simulink model "VELOmodel_i2pacl_steps"  (R2021b)
settings: Solver=ode23t  StartTime=0  StopTime=15000  FixedStep=0.001  MaxStep=0.1  RelTol=1e-6  AbsTol=1e-3  EnableMultiTasking=on
values from neighbouring files (symbols this model uses):
  CO2PropertyTables =     [CO2properties.mat]
  I_conductivity = 0.033    [simscape_paramaters_testing.m]
  initTemp = 20+273.15    (= 293.15)    [simscape_paramaters_testing.m]
  pump_volume = 9.5e-6    (= 9.5e-06)    [simscape_paramaters_testing.m]
  quater_diameter = 6.35/1000    (= 0.00635)    [simscape_paramaters_testing.m]
  quater_wall_thickness = 0.89/1000    (= 0.00089)    [simscape_paramaters_testing.m]
  SS_density = 8000    [simscape_paramaters_testing.m]
  swep_length = swep_area/(2*pi*swep_radius)    (= 6868.79228081)    [simscape_paramaters_testing.m]
  swep_radius = 3.8    [simscape_paramaters_testing.m]
  T_ambient = 273.15+20    (= 293.15)    [simscape_paramaters_testing.m]
  t_start = 3000+t_cool    (= 5000)    [simscape_paramaters_testing.m]
  TL_length = 10    [simscape_paramaters_testing.m]
  TL_supply_diameter = 0.005    [simscape_paramaters_testing.m]
libraries: fl_lib x99, nesl_utility x20, SimscapeFluids_lib x1, slpidlib x1
(part 2 of 2)

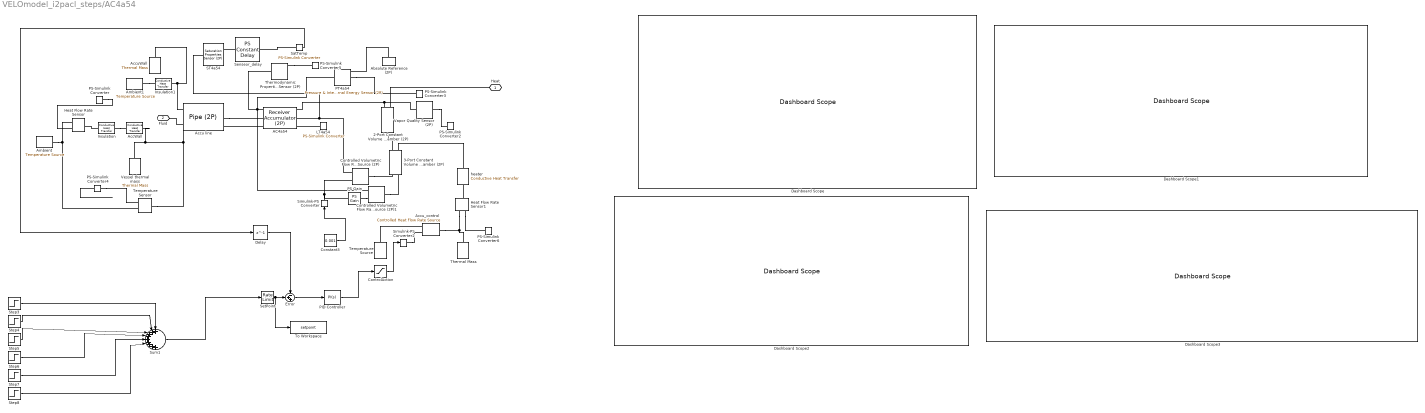
== system VELOmodel_i2pacl_steps/AC4a54 ==
  2-Port Constant Volume Chamber (2P) : fl_lib/Two-Phase Fluid/Elements/2-Port Constant Volume Chamber (2P)  volume=1 l  area_A=1 m^2  area_B=1 m^2  energy_spec=foundation.enum.energy_spec.void_fraction  p_init=initPressure MPa  T_init=initTemp K  x_init=0.5  alpha_init=0.7  h_init=1500 kJ/kg  u_init=1500 kJ/kg  time_constant=0.1 s
      settings: SourceProductBaseCode=SS  InternalSimscapePortConfiguration="{\"Bottom\":[],\"Left\":[{\"id\":\"A\",\"label\":\"A\",\"type\":\"foundation.two_phase_fluid.two_phase_fluid\"},{\"id\":\"H\",\"label\":\"H\",\"type\":\"foundation.thermal.thermal\"}],\"Right\":[{\"id\":\"B\",\"label\":\"B\",\"type\":\"foundation.two_phase_fluid.two_phase_fluid\"}],\"Top\":[]}"
  3-Port Constant Volume Chamber (2P) : fl_lib/Two-Phase Fluid/Elements/3-Port Constant Volume Chamber (2P)  volume=2 l  area_A=1 m^2  area_B=1 m^2  area_C=1 m^2  energy_spec=foundation.enum.energy_spec.void_fraction  p_init=initPressure MPa  T_init=initTemp K  x_init=0.5  alpha_init=0.7  h_init=1500 kJ/kg  u_init=1500 kJ/kg  time_constant=0.1 s
      settings: SourceProductBaseCode=SS  InternalSimscapePortConfiguration="{\"Bottom\":[],\"Left\":[{\"id\":\"A\",\"label\":\"A\",\"type\":\"foundation.two_phase_fluid.two_phase_fluid\"},{\"id\":\"H\",\"label\":\"H\",\"type\":\"foundation.thermal.thermal\"}],\"Right\":[{\"id\":\"B\",\"label\":\"B\",\"type\":\"foundation.two_phase_fluid.two_phase_fluid\"},{\"id\":\"C\",\"label\":\"C\",\"type\":\"foundation.two_phase_fluid.two_phase_fluid\"}],\"Top\":[]}"
  AC4a54 : SimscapeFluids_lib/Two-Phase Fluid/Tanks & Accumulators/Receiver Accumulator (2P)  volume=Acc_volume l  area_AV=1 m^2  area_BV=1 m^2  area_AL=quater_area m^2  area_BL=1 m^2  V_frac_error=simscape.enum.assert.action.none  V_frac_min=0.05  V_frac_max=0.95  V_frac_smooth=0.05  p_crit_error=simscape.enum.assert.action.warn  hc_vap=20 W/(m^2*K)  hc_liq=100 W/(m^2*K)  surface_area=0.5 m^2  receiver_accumulator_energy_spec=fluids.two_phase_fluid.enum.receiver_accumulator_energy_spec.volume_fraction  p_init=initPressure MPa  T_init=initTemp K  M_frac_init=0.5  V_frac_init=0.3  h_init=1500 kJ/kg  u_init=1500 kJ/kg  tau_vap_cond=1 s
      settings: SourceProductBaseCode=SH  InternalSimscapePortConfiguration="{\"Bottom\":[],\"Left\":[{\"id\":\"AV\",\"label\":\"AV\",\"type\":\"foundation.two_phase_fluid.two_phase_fluid\"},{\"id\":\"AL\",\"label\":\"AL\",\"type\":\"foundation.two_phase_fluid.two_phase_fluid\"},{\"id\":\"H\",\"label\":\"H\",\"type\":\"foundation.thermal.thermal\"}],\"Right\":[{\"id\":\"BV\",\"label\":\"BV\",\"type\":\"foundation.two_phase_fluid.two_phase_fluid\"},{\"id\":\"BL\",\"label\":\"BL\",\"type\":\"foundation.two_phase_fluid.two_phase_fluid\"},{\"id\":\"L\",\"label\":\"L\",\"type\":\"output\"}],\"Top\":[]}"
  Absolute Reference (2P) : fl_lib/Two-Phase Fluid/Elements/Absolute Reference (2P)
      settings: SourceProductBaseCode=SS
  AccWall : fl_lib/Thermal/Thermal Elements/Conductive Heat Transfer  area=I_area m^2  thickness=Acc_thickness m  th_cond=SS_conductivity W/(m*K)  T_specify=off  T_priority=None  T=0 K  T_nominal_specify=off  T_nominal_unit=K  T_nominal_value=1  Q_specify=off  Q_priority=None  Q=0 W  Q_nominal_specify=off  Q_nominal_unit=W  Q_nominal_value=1
  Accu line : fl_lib/Two-Phase Fluid/Elements/Pipe (2P)  length=0.5 m  area=quater_area m^2  Dh=quater_diameter m  length_add=0.1 m  roughness=15e-6 m  Re_lam=2000  Re_tur=4000  shape_factor=64  Nu_lam=3.66  inertia=simscape.enum.onoff.off  energy_spec=foundation.enum.energy_spec.void_fraction  p_init=initPressure MPa  T_init=initTemp K  x_init=0  alpha_init=voidFrac  h_init=1500 kJ/kg  u_init=1500 kJ/kg  mdot_init=0 kg/s  time_constant=0.1 s
      settings: SourceProductBaseCode=SS  InternalSimscapePortConfiguration="{\"Bottom\":[],\"Left\":[{\"id\":\"A\",\"label\":\"A\",\"type\":\"foundation.two_phase_fluid.two_phase_fluid\"},{\"id\":\"H\",\"label\":\"H\",\"type\":\"foundation.thermal.thermal\"}],\"Right\":[{\"id\":\"B\",\"label\":\"B\",\"type\":\"foundation.two_phase_fluid.two_phase_fluid\"}],\"Top\":[]}"
  AccuWall : fl_lib/Thermal/Thermal Elements/Thermal Mass  mass=0.5 kg  sp_heat=SS_specific_heat J/(K*kg)  T_specify=on  T_priority=High  T=initTemp K  T_nominal_specify=off  T_nominal_unit=K  T_nominal_value=1  Q_specify=off  Q_priority=None  Q=0 W  Q_nominal_specify=off  Q_nominal_unit=W  Q_nominal_value=1
  Accu_control : fl_lib/Thermal/Thermal Sources/Controlled Heat Flow Rate Source
  Ambient : fl_lib/Thermal/Thermal Sources/Temperature Source  temperature=T_ambient K
  Ambient1 : fl_lib/Thermal/Thermal Sources/Temperature Source  temperature=T_ambient K
  Constant3 : Constant  Value=0.001
  ControlAction : Saturate  UpperLimit=1000  LowerLimit=-1000
  Controlled Volumetric Flow Rate Source (2P) : fl_lib/Two-Phase Fluid/Sources/Controlled Volumetric Flow Rate Source (2P)  power_spec=foundation.enum.power_spec.none  area_A=1 m^2  area_B=1 m^2
      settings: SourceProductBaseCode=SS  InternalSimscapePortConfiguration="{\"Bottom\":[],\"Left\":[{\"id\":\"A\",\"label\":\"A\",\"type\":\"foundation.two_phase_fluid.two_phase_fluid\"},{\"id\":\"V\",\"label\":\"V\",\"type\":\"input\"}],\"Right\":[{\"id\":\"B\",\"label\":\"B\",\"type\":\"foundation.two_phase_fluid.two_phase_fluid\"}],\"Top\":[]}"
  Controlled Volumetric Flow Rate Source (2P)1 : fl_lib/Two-Phase Fluid/Sources/Controlled Volumetric Flow Rate Source (2P)  power_spec=foundation.enum.power_spec.none  area_A=1 m^2  area_B=1 m^2
      settings: SourceProductBaseCode=SS  InternalSimscapePortConfiguration="{\"Bottom\":[],\"Left\":[{\"id\":\"A\",\"label\":\"A\",\"type\":\"foundation.two_phase_fluid.two_phase_fluid\"},{\"id\":\"V\",\"label\":\"V\",\"type\":\"input\"}],\"Right\":[{\"id\":\"B\",\"label\":\"B\",\"type\":\"foundation.two_phase_fluid.two_phase_fluid\"}],\"Top\":[]}"
  Dashboard Scope{,1..3} (4 alike) : DashboardScope
  Delay : Delay  DelayLength=1  InitialCondition=initTemp+5.35
  Error : Sum  Inputs=-++
  Heat Flow Rate Sensor : fl_lib/Thermal/Thermal Sensors/Heat Flow Rate Sensor
      settings: SourceProductBaseCode=SS
  Heat Flow Rate Sensor1 : fl_lib/Thermal/Thermal Sensors/Heat Flow Rate Sensor
      settings: SourceProductBaseCode=SS
  Insulation : fl_lib/Thermal/Thermal Elements/Conductive Heat Transfer  area=I_area m^2  thickness=I_thickness m  th_cond=I_conductivity*4 W/(m*K)  T_specify=off  T_priority=None  T=0 K  T_nominal_specify=off  T_nominal_unit=K  T_nominal_value=1  Q_specify=off  Q_priority=None  Q=0 W  Q_nominal_specify=off  Q_nominal_unit=W  Q_nominal_value=1
  Insulation1 : fl_lib/Thermal/Thermal Elements/Conductive Heat Transfer  area=pi*quater_diameter*1 m^2  thickness=I_thickness m  th_cond=I_conductivity W/(m*K)  T_specify=off  T_priority=None  T=0 K  T_nominal_specify=off  T_nominal_unit=K  T_nominal_value=1  Q_specify=off  Q_priority=None  Q=0 W  Q_nominal_specify=off  Q_nominal_unit=W  Q_nominal_value=1
  LT4a54 : nesl_utility/PS-Simulink Converter  PhysicalDomain=network_engine_domain  SubClassName=ps_output  LeftPortType=input  RightPortType=output  PseudoPeriodic=off  Frequencies=[]  Unit=inherit  AffineConversion=off
      settings: SourceProductBaseCode=PW,SS
  PID Controller : slpidlib/PID Controller  Controller=PI  Form=Ideal  TimeDomain=Continuous-time  UseExternalTs=off  SampleTime=-1  IntegratorMethod=Forward Euler  FilterMethod=Forward Euler  ControllerParametersSource=internal  P=711  I=1/186  D=0  UseFilter=on  N=100  TunerSelectOption=Transfer Function Based (PID Tuner App)  InitialConditionSource=internal  InitialConditionForIntegrator=0  InitialConditionForFilter=0  DifferentiatorICPrevScaledInput=0  ExternalReset=none  TrackingMode=off  Kt=1  LimitOutput=on  SatLimitsSource=internal  UpperSaturationLimit=1000  LowerSaturationLimit=-1000  LinearizeAsGain=on  AntiWindupMode=clamping  Kb=1  POutMin=[]  POutMax=[]  IOutMin=[]  IOutMax=[]  DOutMin=[]  DOutMax=[]  NOutMin=[]  NOutMax=[]  SumOutMin=[]  SumOutMax=[]  SaturationOutMin=[]  SaturationOutMax=[]  PParamMin=[]  PParamMax=[]  IParamMin=[]  IParamMax=[]  DParamMin=[]  DParamMax=[]  NParamMin=[]  NParamMax=[]  KbParamMin=[]  KbParamMax=[]  KtParamMin=[]  KtParamMax=[]  KbOutMin=[]  KbOutMax=[]  KtOutMin=[]  KtOutMax=[]  IntegratorOutMin=[]  IntegratorOutMax=[]  FilterOutMin=[]  FilterOutMax=[]  SumI1OutMin=[]  SumI1OutMax=[]  SumI2OutMin=[]  SumI2OutMax=[]  SumI3OutMin=[]  SumI3OutMax=[]  SumI4OutMin=[]  SumI4OutMax=[]  SumDOutMin=[]  SumDOutMax=[]  DifferentiatorOutMin=[]  DifferentiatorOutMax=[]  FilterDiffOutCoefMin=[]  FilterDiffOutCoefMax=[]  ReciprocalOutMin=[]  ReciprocalOutMax=[]  SumDenOutMin=[]  SumDenOutMax=[]  SumNumOutMin=[]  SumNumOutMax=[]  DivideOutMin=[]  DivideOutMax=[]  UdiffTsProdOutMin=[]  UdiffTsProdOutMax=[]  NTsProdOutMin=[]  NTsProdOutMax=[]  UintegralTsProdOutMin=[]  UintegralTsProdOutMax=[]  UngainTsProdOutMin=[]  UngainTsProdOutMax=[]  IntegratorContinuousStateAttributes=''  IntegratorStateMustResolveToSignalObject=off  IntegratorRTWStateStorageClass=Auto  FilterContinuousStateAttributes=''  FilterStateMustResolveToSignalObject=off  FilterRTWStateStorageClass=Auto  ParallelPVariant=Passthrough  IdealPVariant=InternalParameters  IVariant=InternalParameters  DVariant=Disabled  IntegratorVariant=Continuous  SatVariant=Enabled  AWVariant=ContClampingIdeal  PCopyVariant=InternalParamsIdeal  TRVariant=Disabled  FdbkBlocksVariant=Forward  IdealPFdbkVariant=Disabled  SatFdbkVariant=Disabled  DerivativeFilterVariant=Disabled  NVariant=Disabled  NCopyVariant=Disabled_SignalSpec  FilterICVariant=Disabled  IntegratorICVariant=InternalICs  ExternalResetVariant=Disabled  TRSumVariant=Passthrough  SumFdbkVariant=Disabled  SumVariant=Sum_PI  TsampFilterVariant=InternalTs  TsampNgainVariant=Passthrough  TsampIntegralVariant=Passthrough  ExternalSaturationOutDataTypeStr=Inherit: Same as second input
  PS Gain : fl_lib/Physical Signals/Functions/PS Gain  gain=10
  PS-Simulink Converter{,2..6} (6 alike) : nesl_utility/PS-Simulink Converter  PhysicalDomain=network_engine_domain  SubClassName=ps_output  LeftPortType=input  RightPortType=output  PseudoPeriodic=off  Frequencies=[]  Unit=inherit  AffineConversion=off
      settings: SourceProductBaseCode=PW,SS
  PT4a54 : fl_lib/Two-Phase Fluid/Sensors/Pressure & Internal Energy Sensor (2P)
      settings: SourceProductBaseCode=SS  InternalSimscapePortConfiguration="{\"Bottom\":[],\"Left\":[{\"id\":\"A\",\"label\":\"A\",\"type\":\"foundation.two_phase_fluid.two_phase_fluid\"}],\"Right\":[{\"id\":\"B\",\"label\":\"B\",\"type\":\"foundation.two_phase_fluid.two_phase_fluid\"},{\"id\":\"P\",\"label\":\"P\",\"type\":\"output\"},{\"id\":\"U\",\"label\":\"U\",\"type\":\"output\"}],\"Top\":[]}"
  ST4a54 : fl_lib/Two-Phase Fluid/Sensors/Saturation Properties Sensor (2P)  pressure_measure=simscape.enum.onoff.off  pressure_check=simscape.enum.assert.action.error  energy_measure=foundation.enum.EnergyMeasurement.Off  density_measure=foundation.enum.DensityMeasurement.Off
      settings: SourceProductBaseCode=SS  InternalSimscapePortConfiguration="{\"Bottom\":[],\"Left\":[{\"id\":\"A\",\"label\":\"A\",\"type\":\"foundation.two_phase_fluid.two_phase_fluid\"}],\"Right\":[{\"id\":\"T_sat_liq\",\"label\":\"TL\",\"type\":\"output\"},{\"id\":\"T_sat_vap\",\"label\":\"TV\",\"type\":\"output\"}],\"Top\":[]}"
  SatTemp : nesl_utility/PS-Simulink Converter  PhysicalDomain=network_engine_domain  SubClassName=ps_output  LeftPortType=input  RightPortType=output  PseudoPeriodic=off  Frequencies=[]  Unit=inherit  AffineConversion=off
      settings: SourceProductBaseCode=PW,SS
  Senseor_delay : fl_lib/Physical Signals/Delays/PS Constant Delay  InputHistory=initTemp K  DelayTime=55 ms
      settings: SourceProductBaseCode=SS  InternalSimscapePortConfiguration="{\"Bottom\":[],\"Left\":[{\"id\":\"U\",\"label\":\"U\",\"type\":\"input\"}],\"Right\":[{\"id\":\"Y\",\"label\":\"Y\",\"type\":\"output\"}],\"Top\":[]}"
  SetPoint : RateLimiter  RisingSlewLimit=1.333/60  FallingSlewLimit=-1.333/60  SampleTimeMode=inherited
  Simulink-PS Converter : nesl_utility/Simulink-PS Converter  PhysicalDomain=network_engine_domain  SubClassName=ps_input  LeftPortType=input  RightPortType=output  PseudoPeriodic=off  Frequencies=[]  NoiseDistribution=none  NoiseParameters=[]  Unit=1  AffineConversion=off  FilteringAndDerivatives=provide  SimscapeFilterOrder=1  InputFilterTimeConstant=0.001  UdotUserProvided=0
      settings: SourceProductBaseCode=PW,SS
  Simulink-PS Converter2 : nesl_utility/Simulink-PS Converter  PhysicalDomain=network_engine_domain  SubClassName=ps_input  LeftPortType=input  RightPortType=output  PseudoPeriodic=off  Frequencies=[]  NoiseDistribution=none  NoiseParameters=[]  Unit=1  AffineConversion=off  FilteringAndDerivatives=provide  SimscapeFilterOrder=1  InputFilterTimeConstant=0.001  UdotUserProvided=0
      settings: SourceProductBaseCode=PW,SS
  Step3 : Step  Time=500  Before=initTemp  After=273.15-25  SampleTime=0
  Step4 : Step  Time=5000  After=10  SampleTime=0
  Step5 : Step  Time=7000  After=10  SampleTime=0
  Step6 : Step  Time=9000  After=10  SampleTime=0
  Step7 : Step  Time=11000  After=10  SampleTime=0
  Step8 : Step  Time=13000  After=10  SampleTime=0
  Sum1 : Sum  Inputs=+++++++++
  Temperature Sensor : fl_lib/Thermal/Thermal Sensors/Temperature Sensor
  Temperature Source : fl_lib/Thermal/Thermal Sources/Temperature Source  temperature=273 K
  Thermal Mass : fl_lib/Thermal/Thermal Elements/Thermal Mass  mass=2 kg  sp_heat=SS_specific_heat J/(K*kg)  T_specify=on  T_priority=High  T=initTemp K  T_nominal_specify=off  T_nominal_unit=K  T_nominal_value=1  Q_specify=off  Q_priority=None  Q=0 W  Q_nominal_specify=off  Q_nominal_unit=W  Q_nominal_value=1
  Thermodynamic Properties Sensor (2P) : fl_lib/Two-Phase Fluid/Sensors/Thermodynamic Properties Sensor (2P)
      settings: SourceProductBaseCode=SS  InternalSimscapePortConfiguration="{\"Bottom\":[],\"Left\":[{\"id\":\"A\",\"label\":\"A\",\"type\":\"foundation.two_phase_fluid.two_phase_fluid\"}],\"Right\":[{\"id\":\"T\",\"label\":\"T\",\"type\":\"output\"},{\"id\":\"H\",\"label\":\"h\",\"type\":\"output\"},{\"id\":\"V\",\"label\":\"v\",\"type\":\"output\"},{\"id\":\"S\",\"label\":\"s\",\"type\":\"output\"}],\"Top\":[]}"
  To Workspace : ToWorkspace  VariableName=setpoint  SaveFormat=Timeseries  SampleTime=-1
  Vapor Quality Sensor (2P) : fl_lib/Two-Phase Fluid/Sensors/Vapor Quality Sensor (2P)  vapor_fraction_spec=foundation.enum.vapor_fraction_spec.quality
      settings: SourceProductBaseCode=SS  InternalSimscapePortConfiguration="{\"Bottom\":[],\"Left\":[{\"id\":\"A\",\"label\":\"A\",\"type\":\"foundation.two_phase_fluid.two_phase_fluid\"}],\"Right\":[{\"id\":\"X\",\"label\":\"X\",\"type\":\"output\"}],\"Top\":[]}"
  Vessel thermal mass : fl_lib/Thermal/Thermal Elements/Thermal Mass  mass=A_mass kg  sp_heat=SS_specific_heat J/(K*kg)  T_specify=on  T_priority=High  T=initTemp K  T_nominal_specify=off  T_nominal_unit=K  T_nominal_value=1  Q_specify=off  Q_priority=None  Q=0 W  Q_nominal_specify=off  Q_nominal_unit=W  Q_nominal_value=1
  heater : fl_lib/Thermal/Thermal Elements/Conductive Heat Transfer  area=0.25 m^2  thickness=0.001 m  th_cond=SS_conductivity W/(m*K)  T_specify=off  T_priority=None  T=0 K  T_nominal_specify=off  T_nominal_unit=K  T_nominal_value=1  Q_specify=off  Q_priority=None  Q=0 W  Q_nominal_specify=off  Q_nominal_unit=W  Q_nominal_value=1
  Heat : PMIOPort  Side=Left
  Fluid : PMIOPort  Port=2  Side=Left
  wires:
  PS-Simulink Converter4/1 -> ?
  SatTemp/1 -> Delay/1
  Constant3/1 -> Simulink-PS Converter/1
  PID Controller/1 -> ControlAction/1
  SetPoint/1 -> To Workspace/1, Error/2
  Error/1 -> PID Controller/1
  Delay/1 -> Error/1
  ControlAction/1 -> Simulink-PS Converter2/1
  Step8/1 -> Sum1/6
  Step7/1 -> Sum1/5
  Step5/1 -> Sum1/3
  Step4/1 -> Sum1/2
  Step6/1 -> Sum1/4
  Sum1/1 -> SetPoint/1
  Step3/1 -> Sum1/1
  connections:
  Vessel thermal mass/LConn1 -- AccWall/RConn1 -- Temperature Sensor/LConn1 -- AC4a54/LConn3
  LT4a54/LConn1 -- AC4a54/RConn3
  AC4a54/LConn1 -- Thermodynamic Properties Sensor (2P)/LConn1 -- PT4a54/LConn1 -- Controlled Volumetric Flow Rate Source (2P)1/LConn1
  Temperature Source/LConn1 -- Accu_control/RConn2
  Vapor Quality Sensor (2P)/RConn1 -- PS-Simulink Converter2/LConn1
  Vapor Quality Sensor (2P)/LConn1 -- 2-Port Constant Volume Chamber (2P)/LConn1 -- AC4a54/RConn1
  Absolute Reference (2P)/LConn1 -- PT4a54/RConn1
  PT4a54/RConn2 -- PS-Simulink Converter3/LConn1
  Controlled Volumetric Flow Rate Source (2P)/LConn1 -- ST4a54/LConn1 -- AC4a54/RConn2
  Controlled Volumetric Flow Rate Source (2P)/LConn2 -- PS Gain/LConn1 -- Simulink-PS Converter/RConn1
  Senseor_delay/LConn1 -- ST4a54/RConn1
  Temperature Sensor/RConn1 -- Ambient/LConn1 -- Heat Flow Rate Sensor/RConn2
  PS-Simulink Converter/LConn1 -- Heat Flow Rate Sensor/RConn1
  PS-Simulink Converter4/LConn1 -- Temperature Sensor/RConn2
  Thermodynamic Properties Sensor (2P)/RConn1 -- PS-Simulink Converter5/LConn1
  Heat Flow Rate Sensor1/RConn2 -- Accu_control/LConn1 -- Thermal Mass/LConn1
  3-Port Constant Volume Chamber (2P)/LConn2 -- heater/RConn1
  Heat Flow Rate Sensor1/LConn1 -- heater/LConn1
  Heat Flow Rate Sensor1/RConn1 -- PS-Simulink Converter6/LConn1
  Simulink-PS Converter2/RConn1 -- Accu_control/RConn1
  Controlled Volumetric Flow Rate Source (2P)/RConn1 -- 3-Port Constant Volume Chamber (2P)/RConn1
  Controlled Volumetric Flow Rate Source (2P)1/RConn1 -- 3-Port Constant Volume Chamber (2P)/RConn2
  PS Gain/RConn1 -- Controlled Volumetric Flow Rate Source (2P)1/LConn2
  3-Port Constant Volume Chamber (2P)/LConn1 -- 2-Port Constant Volume Chamber (2P)/RConn1
  Heat/RConn1 -- 2-Port Constant Volume Chamber (2P)/LConn2
  SatTemp/LConn1 -- Senseor_delay/RConn1
  Accu line/RConn1 -- AC4a54/LConn2
  Accu line/LConn1 -- Fluid/RConn1
  Ambient1/LConn1 -- Insulation1/LConn1
  Insulation1/RConn1 -- AccuWall/LConn1 -- Accu line/LConn2
  Insulation/RConn1 -- AccWall/LConn1
  Insulation/LConn1 -- Heat Flow Rate Sensor/LConn1

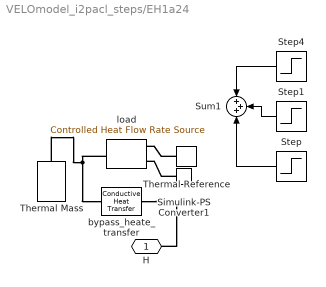
== system VELOmodel_i2pacl_steps/EH1a24 ==
  Simulink-PS Converter1 : nesl_utility/Simulink-PS Converter  PhysicalDomain=network_engine_domain  SubClassName=ps_input  LeftPortType=input  RightPortType=output  PseudoPeriodic=off  Frequencies=[]  NoiseDistribution=none  NoiseParameters=[]  Unit=1  AffineConversion=off  FilteringAndDerivatives=provide  SimscapeFilterOrder=1  InputFilterTimeConstant=0.001  UdotUserProvided=0
      settings: SourceProductBaseCode=PW,SS
  Step : Step  Time=t_start+140  After=400  SampleTime=0
  Step1 : Step  Time=t_start  After=110  SampleTime=0
  Step4 : Step  Time=t_start+5130  After=-510  SampleTime=0
  Sum1 : Sum  Inputs=+++
  Thermal Mass : fl_lib/Thermal/Thermal Elements/Thermal Mass  mass=10 kg  sp_heat=SS_specific_heat J/(K*kg)  T_specify=on  T_priority=High  T=initTemp K  T_nominal_specify=off  T_nominal_unit=K  T_nominal_value=1  Q_specify=off  Q_priority=None  Q=0 W  Q_nominal_specify=off  Q_nominal_unit=W  Q_nominal_value=1
  Thermal Reference : fl_lib/Thermal/Thermal Elements/Thermal Reference
  bypass_heate_transfer : fl_lib/Thermal/Thermal Elements/Conductive Heat Transfer  area=0.25 m^2  thickness=0.001 m  th_cond=SS_conductivity W/(m*K)  T_specify=off  T_priority=None  T=0 K  T_nominal_specify=off  T_nominal_unit=K  T_nominal_value=1  Q_specify=off  Q_priority=None  Q=0 W  Q_nominal_specify=off  Q_nominal_unit=W  Q_nominal_value=1
  load : fl_lib/Thermal/Thermal Sources/Controlled Heat Flow Rate Source
  H : PMIOPort  Side=Right
  wires:
  Step1/1 -> Sum1/2
  Step4/1 -> Sum1/1
  Step/1 -> Sum1/3
  connections:
  Simulink-PS Converter1/RConn1 -- load/RConn1
  load/LConn1 -- Thermal Mass/LConn1 -- bypass_heate_transfer/LConn1
  Thermal Reference/LConn1 -- load/RConn2
  bypass_heate_transfer/RConn1 -- H/RConn1

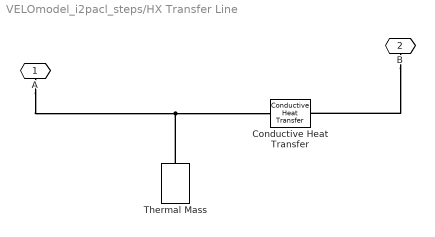
== system VELOmodel_i2pacl_steps/HX Transfer Line ==
  Conductive Heat Transfer : fl_lib/Thermal/Thermal Elements/Conductive Heat Transfer  area=TL_length*pi*TL_supply_diameter m^2  thickness=TL_wall_thickness m  th_cond=SS_conductivity W/(m*K)  T_specify=off  T_priority=None  T=0 K  T_nominal_specify=off  T_nominal_unit=K  T_nominal_value=1  Q_specify=off  Q_priority=None  Q=0 W  Q_nominal_specify=off  Q_nominal_unit=W  Q_nominal_value=1
  Thermal Mass : fl_lib/Thermal/Thermal Elements/Thermal Mass  mass=TL_length*pi*quater_diameter*quater_wall_thickness*SS_density kg  sp_heat=SS_specific_heat J/(K*kg)  T_specify=off  T_priority=High  T=300 K  T_nominal_specify=off  T_nominal_unit=K  T_nominal_value=1  Q_specify=off  Q_priority=None  Q=0 W  Q_nominal_specify=off  Q_nominal_unit=W  Q_nominal_value=1
  A : PMIOPort  Side=Left
  B : PMIOPort  Port=2  Side=Right
  connections:
  B/RConn1 -- Conductive Heat Transfer/RConn1
  A/RConn1 -- Conductive Heat Transfer/LConn1 -- Thermal Mass/LConn1

== system VELOmodel_i2pacl_steps/HX4a54b ==
  Conductive Heat Transfer : fl_lib/Thermal/Thermal Elements/Conductive Heat Transfer  area=hx_sa m^2  thickness=quater_wall_thickness m  th_cond=SS_conductivity W/(m*K)  T_specify=off  T_priority=None  T=0 K  T_nominal_specify=off  T_nominal_unit=K  T_nominal_value=1  Q_specify=off  Q_priority=None  Q=0 W  Q_nominal_specify=off  Q_nominal_unit=W  Q_nominal_value=1
  Thermal Mass : fl_lib/Thermal/Thermal Elements/Thermal Mass  mass=hx_mass kg  sp_heat=SS_specific_heat J/(K*kg)  T_specify=off  T_priority=High  T=300 K  T_nominal_specify=off  T_nominal_unit=K  T_nominal_value=1  Q_specify=off  Q_priority=None  Q=0 W  Q_nominal_specify=off  Q_nominal_unit=W  Q_nominal_value=1
  A : PMIOPort  Side=Left
  B : PMIOPort  Port=2  Side=Right
  connections:
  B/RConn1 -- Conductive Heat Transfer/RConn1
  A/RConn1 -- Conductive Heat Transfer/LConn1 -- Thermal Mass/LConn1

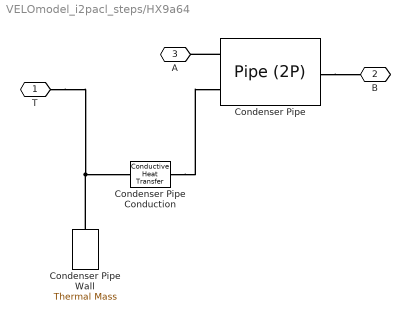
== system VELOmodel_i2pacl_steps/HX9a64 ==
  Condenser Pipe Wall : fl_lib/Thermal/Thermal Elements/Thermal Mass  mass=swep_mass kg  sp_heat=SS_specific_heat J/(K*kg)  T_specify=on  T_priority=Low  T=initTemp K  T_nominal_specify=off  T_nominal_unit=K  T_nominal_value=1  Q_specify=off  Q_priority=None  Q=0 W  Q_nominal_specify=off  Q_nominal_unit=W  Q_nominal_value=1
  Condenser Pipe : fl_lib/Two-Phase Fluid/Elements/Pipe (2P)  length=swep_length mm  area=swep_cross_section mm^2  Dh=2*swep_radius mm  length_add=0.1*swep_length m  roughness=1.5e-5 m  Re_lam=2e+3  Re_tur=4e+3  shape_factor=64  Nu_lam=3.66  inertia=simscape.enum.onoff.off  energy_spec=foundation.enum.energy_spec.void_fraction  p_init=initPressure MPa  T_init=initTemp K  x_init=0  alpha_init=voidFrac  h_init=1500 kJ/kg  u_init=1500 kJ/kg  mdot_init=0 kg/s  time_constant=0.1 s
      settings: SourceProductBaseCode=SS  InternalSimscapePortConfiguration="{\"Bottom\":[],\"Left\":[{\"id\":\"A\",\"label\":\"A\",\"type\":\"foundation.two_phase_fluid.two_phase_fluid\"},{\"id\":\"H\",\"label\":\"H\",\"type\":\"foundation.thermal.thermal\"}],\"Right\":[{\"id\":\"B\",\"label\":\"B\",\"type\":\"foundation.two_phase_fluid.two_phase_fluid\"}],\"Top\":[]}"
  Condenser Pipe Conduction : fl_lib/Thermal/Thermal Elements/Conductive Heat Transfer  area=swep_area mm^2  thickness=swep_thickness m  th_cond=SS_conductivity W/(m*K)  T_specify=off  T_priority=None  T=0 K  T_nominal_specify=off  T_nominal_unit=K  T_nominal_value=1  Q_specify=off  Q_priority=None  Q=0 W  Q_nominal_specify=off  Q_nominal_unit=W  Q_nominal_value=1
  T : PMIOPort  Side=Left
  B : PMIOPort  Port=2  Side=Left
  A : PMIOPort  Port=3  Side=Right
  connections:
  Condenser Pipe/LConn1 -- A/RConn1
  Condenser Pipe/RConn1 -- B/RConn1
  Condenser Pipe Conduction/LConn1 -- Condenser Pipe/LConn2
  Condenser Pipe Wall/LConn1 -- T/RConn1 -- Condenser Pipe Conduction/RConn1

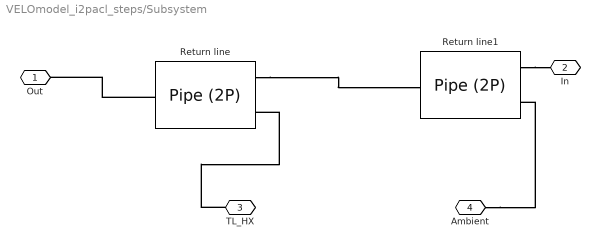
== system VELOmodel_i2pacl_steps/Subsystem ==
  Return line : fl_lib/Two-Phase Fluid/Elements/Pipe (2P)  length=TL_length/2 m  area=TL_return_cross_section m^2  Dh=TL_return_diameter m  length_add=0.1 m  roughness=15e-6 m  Re_lam=2000  Re_tur=4000  shape_factor=64  Nu_lam=3.66  inertia=simscape.enum.onoff.off  energy_spec=foundation.enum.energy_spec.void_fraction  p_init=initPressure MPa  T_init=initTemp K  x_init=0  alpha_init=voidFrac  h_init=1500 kJ/kg  u_init=1500 kJ/kg  mdot_init=0 kg/s  time_constant=0.1 s
      settings: SourceProductBaseCode=SS  InternalSimscapePortConfiguration="{\"Bottom\":[],\"Left\":[{\"id\":\"A\",\"label\":\"A\",\"type\":\"foundation.two_phase_fluid.two_phase_fluid\"},{\"id\":\"H\",\"label\":\"H\",\"type\":\"foundation.thermal.thermal\"}],\"Right\":[{\"id\":\"B\",\"label\":\"B\",\"type\":\"foundation.two_phase_fluid.two_phase_fluid\"}],\"Top\":[]}"
  Return line1 : fl_lib/Two-Phase Fluid/Elements/Pipe (2P)  length=TL_length/2 m  area=TL_return_cross_section m^2  Dh=TL_return_diameter m  length_add=0.1 m  roughness=15e-6 m  Re_lam=2000  Re_tur=4000  shape_factor=64  Nu_lam=3.66  inertia=simscape.enum.onoff.off  energy_spec=foundation.enum.energy_spec.void_fraction  p_init=initPressure MPa  T_init=initTemp K  x_init=0  alpha_init=voidFrac  h_init=1500 kJ/kg  u_init=1500 kJ/kg  mdot_init=0 kg/s  time_constant=0.1 s
      settings: SourceProductBaseCode=SS  InternalSimscapePortConfiguration="{\"Bottom\":[],\"Left\":[{\"id\":\"A\",\"label\":\"A\",\"type\":\"foundation.two_phase_fluid.two_phase_fluid\"},{\"id\":\"H\",\"label\":\"H\",\"type\":\"foundation.thermal.thermal\"}],\"Right\":[{\"id\":\"B\",\"label\":\"B\",\"type\":\"foundation.two_phase_fluid.two_phase_fluid\"}],\"Top\":[]}"
  Out : PMIOPort  Side=Left
  In : PMIOPort  Port=2  Side=Right
  TL_HX : PMIOPort  Port=3  Side=Right
  Ambient : PMIOPort  Port=4  Side=Right
  connections:
  Return line/RConn1 -- Out/RConn1
  Return line1/LConn1 -- In/RConn1
  Return line/LConn1 -- Return line1/RConn1
  Ambient/RConn1 -- Return line1/LConn2
  TL_HX/RConn1 -- Return line/LConn2

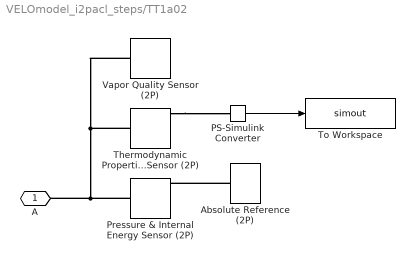
== system VELOmodel_i2pacl_steps/TT1a02 ==
  Absolute Reference (2P) : fl_lib/Two-Phase Fluid/Elements/Absolute Reference (2P)
      settings: SourceProductBaseCode=SS
  PS-Simulink Converter : nesl_utility/PS-Simulink Converter  PhysicalDomain=network_engine_domain  SubClassName=ps_output  LeftPortType=input  RightPortType=output  PseudoPeriodic=off  Frequencies=[]  Unit=inherit  AffineConversion=off
      settings: SourceProductBaseCode=PW,SS
  Pressure & Internal Energy Sensor (2P) : fl_lib/Two-Phase Fluid/Sensors/Pressure & Internal Energy Sensor (2P)
      settings: SourceProductBaseCode=SS  InternalSimscapePortConfiguration="{\"Bottom\":[],\"Left\":[{\"id\":\"A\",\"label\":\"A\",\"type\":\"foundation.two_phase_fluid.two_phase_fluid\"}],\"Right\":[{\"id\":\"B\",\"label\":\"B\",\"type\":\"foundation.two_phase_fluid.two_phase_fluid\"},{\"id\":\"P\",\"label\":\"P\",\"type\":\"output\"},{\"id\":\"U\",\"label\":\"U\",\"type\":\"output\"}],\"Top\":[]}"
  Thermodynamic Properties Sensor (2P) : fl_lib/Two-Phase Fluid/Sensors/Thermodynamic Properties Sensor (2P)
      settings: SourceProductBaseCode=SS  InternalSimscapePortConfiguration="{\"Bottom\":[],\"Left\":[{\"id\":\"A\",\"label\":\"A\",\"type\":\"foundation.two_phase_fluid.two_phase_fluid\"}],\"Right\":[{\"id\":\"T\",\"label\":\"T\",\"type\":\"output\"},{\"id\":\"H\",\"label\":\"h\",\"type\":\"output\"},{\"id\":\"V\",\"label\":\"v\",\"type\":\"output\"},{\"id\":\"S\",\"label\":\"s\",\"type\":\"output\"}],\"Top\":[]}"
  To Workspace : ToWorkspace  VariableName=simout  SaveFormat=Timeseries  SampleTime=-1
  Vapor Quality Sensor (2P) : fl_lib/Two-Phase Fluid/Sensors/Vapor Quality Sensor (2P)  vapor_fraction_spec=foundation.enum.vapor_fraction_spec.quality
      settings: SourceProductBaseCode=SS  InternalSimscapePortConfiguration="{\"Bottom\":[],\"Left\":[{\"id\":\"A\",\"label\":\"A\",\"type\":\"foundation.two_phase_fluid.two_phase_fluid\"}],\"Right\":[{\"id\":\"X\",\"label\":\"X\",\"type\":\"output\"}],\"Top\":[]}"
  A : PMIOPort  Side=Left
  wires:
  PS-Simulink Converter/1 -> To Workspace/1
  connections:
  Thermodynamic Properties Sensor (2P)/LConn1 -- Vapor Quality Sensor (2P)/LConn1 -- A/RConn1 -- Pressure & Internal Energy Sensor (2P)/LConn1
  Absolute Reference (2P)/LConn1 -- Pressure & Internal Energy Sensor (2P)/RConn1
  Thermodynamic Properties Sensor (2P)/RConn1 -- PS-Simulink Converter/LConn1

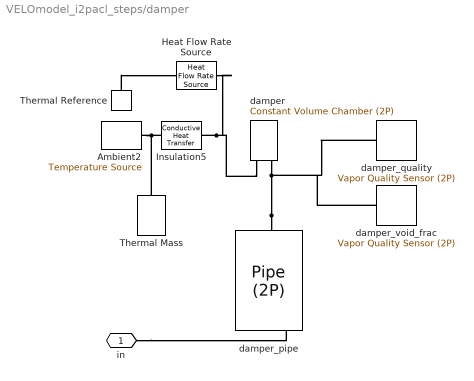
== system VELOmodel_i2pacl_steps/damper ==
  Ambient2 : fl_lib/Thermal/Thermal Sources/Temperature Source  temperature=T_ambient+6 K
  Heat Flow Rate Source : fl_lib/Thermal/Thermal Sources/Heat Flow Rate Source  heat_flow=150 W
      settings: SourceProductBaseCode=SS  InternalSimscapePortConfiguration="{\"Bottom\":[],\"Left\":[{\"id\":\"B\",\"label\":\"B\",\"type\":\"foundation.thermal.thermal\"}],\"Right\":[{\"id\":\"A\",\"label\":\"A\",\"type\":\"foundation.thermal.thermal\"}],\"Top\":[]}"
  Insulation5 : fl_lib/Thermal/Thermal Elements/Conductive Heat Transfer  area=0.001 m^2  thickness=0.007 m  th_cond=SS_conductivity W/(m*K)  T_specify=off  T_priority=None  T=0 K  T_nominal_specify=off  T_nominal_unit=K  T_nominal_value=1  Q_specify=off  Q_priority=None  Q=0 W  Q_nominal_specify=off  Q_nominal_unit=W  Q_nominal_value=1
  Thermal Mass : fl_lib/Thermal/Thermal Elements/Thermal Mass  mass=1 kg  sp_heat=SS_specific_heat J/(K*kg)  T_specify=on  T_priority=Low  T=T_ambient K  T_nominal_specify=off  T_nominal_unit=K  T_nominal_value=1  Q_specify=off  Q_priority=None  Q=0 W  Q_nominal_specify=off  Q_nominal_unit=W  Q_nominal_value=1
  Thermal Reference : fl_lib/Thermal/Thermal Elements/Thermal Reference
  damper : fl_lib/Two-Phase Fluid/Elements/Constant Volume Chamber (2P)  volume=0.6 l  area_A=quater_area m^2  energy_spec=foundation.enum.energy_spec.temperature  p_init=initPressure MPa  T_init=T_ambient K  x_init=0.5  alpha_init=1  h_init=1500 kJ/kg  u_init=1500 kJ/kg  time_constant=0.1 s
      settings: SourceProductBaseCode=SS  InternalSimscapePortConfiguration="{\"Bottom\":[],\"Left\":[{\"id\":\"A\",\"label\":\"A\",\"type\":\"foundation.two_phase_fluid.two_phase_fluid\"},{\"id\":\"H\",\"label\":\"H\",\"type\":\"foundation.thermal.thermal\"}],\"Right\":[],\"Top\":[]}"
  damper_pipe : fl_lib/Two-Phase Fluid/Elements/Pipe (2P)  length=0.2 m  area=quater_area m^2  Dh=quater_diameter m  length_add=0.1 m  roughness=15e-6 m  Re_lam=2000  Re_tur=4000  shape_factor=64  Nu_lam=3.66  inertia=simscape.enum.onoff.off  energy_spec=foundation.enum.energy_spec.void_fraction  p_init=initPressure MPa  T_init=initTemp K  x_init=0  alpha_init=voidFrac  h_init=1500 kJ/kg  u_init=1500 kJ/kg  mdot_init=0 kg/s  time_constant=0.1 s
      settings: SourceProductBaseCode=SS  InternalSimscapePortConfiguration="{\"Bottom\":[],\"Left\":[{\"id\":\"A\",\"label\":\"A\",\"type\":\"foundation.two_phase_fluid.two_phase_fluid\"},{\"id\":\"H\",\"label\":\"H\",\"type\":\"foundation.thermal.thermal\"}],\"Right\":[{\"id\":\"B\",\"label\":\"B\",\"type\":\"foundation.two_phase_fluid.two_phase_fluid\"}],\"Top\":[]}"
  damper_quality : fl_lib/Two-Phase Fluid/Sensors/Vapor Quality Sensor (2P)  vapor_fraction_spec=foundation.enum.vapor_fraction_spec.quality
      settings: SourceProductBaseCode=SS  InternalSimscapePortConfiguration="{\"Bottom\":[],\"Left\":[{\"id\":\"A\",\"label\":\"A\",\"type\":\"foundation.two_phase_fluid.two_phase_fluid\"}],\"Right\":[{\"id\":\"X\",\"label\":\"X\",\"type\":\"output\"}],\"Top\":[]}"
  damper_void_frac : fl_lib/Two-Phase Fluid/Sensors/Vapor Quality Sensor (2P)  vapor_fraction_spec=foundation.enum.vapor_fraction_spec.void_fraction
      settings: SourceProductBaseCode=SS  InternalSimscapePortConfiguration="{\"Bottom\":[],\"Left\":[{\"id\":\"A\",\"label\":\"A\",\"type\":\"foundation.two_phase_fluid.two_phase_fluid\"}],\"Right\":[{\"id\":\"X\",\"label\":\"X\",\"type\":\"output\"}],\"Top\":[]}"
  in : PMIOPort  Side=Left
  connections:
  Insulation5/LConn1 -- Thermal Mass/LConn1 -- Ambient2/LConn1
  Insulation5/RConn1 -- damper/LConn2 -- Heat Flow Rate Source/LConn1
  damper_pipe/RConn1 -- damper/LConn1 -- damper_quality/LConn1 -- damper_void_frac/LConn1
  in/RConn1 -- damper_pipe/LConn1
  Thermal Reference/LConn1 -- Heat Flow Rate Source/RConn1
